simulink model "sm_forklift"  (R2026a)
settings: Solver=daessc  StopTime=stopTime
undefined symbols (not defined in the file): activeTestCmds, ForkliftParams, Ideal, X, Y, Z
libraries: sm_lib x153, nesl_utility x33, fl_lib x12, sm_forklift_lib x4, sdl_lib x3, Camera_Frame_Definitions x1, ee_lib x1, grid_element x1, simulink_extras x1, SignalEditorBlockLib x1
(part 1 of 7)
Description:
  | Copyright 2025-2026 The MathWorks, Inc.
settings Model: Creator=gabri  LastModifiedBy=smiller
settings DataIOCC: ExternalInput=[t,u]  SignalLoggingName=logsout_sm_forklift
settings SimscapeCC: SimscapeNominalValues="[{\"value\":\"1\",\"unit\":\"A\"},{\"value\":\"1\",\"unit\":\"bar\"},{\"value\":\"1\",\"unit\":\"cm^2\"},{\"value\":\"1\",\"unit\":\"cm^3/s\"},{\"value\":\"1\",\"unit\":\"kJ/kg\"},{\"value\":\"1\",\"unit\":\"kW\"},{\"value\":\"1\",\"unit\":\"l\"},{\"value\":\"1\",\"unit\":\"N\"},{\"value\":\"1\",\"unit\":\"N*m\"},{\"value\":\"1\",\"unit\":\"V\"}]"  SimscapeLogName=simlog_sm_forklift  SimscapeLogLimitData=off  SimscapeLogDataHistory=5000.0
settings DiagnosticsConfigSet: SimMechanicsConflictingReferenceFrames=none
settings ExplorerConfigSet: InternalSimMechanicsExplorerSettings="<ExplorerConfiguration><canonicalview>default</canonicalview><AnimationSetting><BasePlaybackSpeed>1.0</BasePlaybackSpeed><PlaybackSpeedFactor>2.0</PlaybackSpeedFactor></AnimationSetting><TilePanel><TileInfo><Tiles Columns=\"2\" Count=\"3\" Rows=\"2\"><Column Weight=\"0.5\"/><Column Weight=\"0.5\"/><Row Weight=\"0.4992\"/><Row Weight=\"0.5008\"/><Tile Height=\"2\" Width=\"1\" X=\"0\" Y=\"0\"/><Tile Height=\"1\" Width=\"1\" X=\"1\" Y=\"0\"/><Tile Height=\"1\" Width=\"1\" X=\"1\" Y=\"1\"/></Tiles></TileInfo><SceneInfo><SceneViewer><BGColor><R>1</R><G>1</G><B>1</B></BGColor><Camera><DoPerspective>on</DoPerspective><Position><X>4.09572120067952739</X><Y>-3.20098882363330972</Y><Z>2.29774941731300508</Z></Position><Center><X>3.34545211978248291</X><Y>-2.5757645895524397</Y><Z>2.08282858684770611</Z></Center><Up><X>-0.16510675539218278</X><Y>0.137588962826818928</Y><Z>0.976631474319820447</Z></Up><ViewLimDist>1</ViewLimDist><YLim>0.466307658154998583</YLim><XLim>0.48985854998100864</XLim></Camera></SceneViewer><SceneViewer><BGColor><R>1</R><G>1</G><B>1</B></BGColor><Camera><DoPerspective>on</DoPerspective><Position><X>0.255721200679526584</X><Y>-0.000988823633308211214</Y><Z>7.19774941731300544</Z></Position><Center><X>0.255721200679526584</X><Y>-0.000988823633308211214</Y><Z>6.19774941731300544</Z></Center><Up><X>0</X><Y>1</Y><Z>0</Z></Up><ViewLimDist>1</ViewLimDist><YLim>0.466307658154998583</YLim><XLim>0.996493077701092966</XLim></Camera></SceneViewer><SceneViewer><BGColor><R>1</R><G>1</G><B>1</B></BGColor><Camera><DoPerspective>on</DoPerspective><Position><X>0.255721200679527028</X><Y>-5.00098882363330866</Y><Z>1.8477494173130049</Z></Position><Center><X>0.255721200679526806</X><Y>-4.00933320629007106</Y><Z>1.71883418705838409</Z></Center><Up><X>-1.38777878078144568e-17</X><Y>0.128915230254620927</Y><Z>0.991655617343237816</Z></Up><ViewLimDist>1</ViewLimDist><YLim>0.466307658154998583</YLim><XLim>0.993092077435901444</XLim></Camera></SceneViewer></SceneInfo></TilePanel><MechEditorPanel><Cameras><Camera><Id>Camera1</Id><Value><Name>Track FixO FR</Name><NativeCamera><PositionTrackingFeature>Camera_Frames.Frame_FixO_FR.R</PositionTrackingFeature><CenterTrackingFeature>Camera_Frames.Frame_FixO_FR.R</CenterTrackingFeature><UpVectorTrackingFeature>Camera_Frames.Frame_FixO_FR.R</UpVectorTrackingFeature><CenterTrackingOrigin>off</CenterTrackingOrigin><CenterTrackingDirection>+X</CenterTrackingDirection><UpVectorTrackingDirection>+Z</UpVectorTrackingDirection></NativeCamera></Value></Camera><Camera><Id>Camera2</Id><Value><Name>Track FixO Right</Name><NativeCamera><PositionTrackingFeature>Camera_Frames.Frame_FixO_Right.R</PositionTrackingFeature><CenterTrackingFeature>Camera_Frames.Frame_FixO_Right.R</CenterTrackingFeature><UpVectorTrackingFeature>Camera_Frames.Frame_FixO_Right.R</UpVectorTrackingFeature><CenterTrackingOrigin>off</CenterTrackingOrigin><CenterTrackingDirection>+X</CenterTrackingDirection><UpVectorTrackingDirection>+Z</UpVectorTrackingDirection></NativeCamera></Value></Camera><Camera><Id>Camera3</Id><Value><Name>Track FixO RR</Name><NativeCamera><PositionTrackingFeature>Camera_Frames.Frame_FixO_RR.R</PositionTrackingFeature><CenterTrackingFeature>Camera_Frames.Frame_FixO_RR.R</CenterTrackingFeature><UpVectorTrackingFeature>Camera_Frames.Frame_FixO_RR.R</UpVectorTrackingFeature><CenterTrackingOrigin>off</CenterTrackingOrigin><CenterTrackingDirection>+X</CenterTrackingDirection><UpVectorTrackingDirection>+Z</UpVectorTrackingDirection></NativeCamera></Value></Camera><Camera><Id>Camera4</Id><Value><Name>Track FixO RL</Name><NativeCamera><PositionTrackingFeature>Camera_Frames.Frame_FixO_RL.R</PositionTrackingFeature><CenterTrackingFeature>Camera_Frames.Frame_FixO_RL.R</CenterTrackingFeature><UpVectorTrackingFeature>Camera_Frames.Frame_FixO_RL.R</UpVectorTrackingFeature><CenterTrackingOrigin>off</CenterTrackingOrigin><CenterTrackingDirection>+X</CenterTrackingDirection><UpVectorTrackingDirection>+Z</UpVectorTrackingDirection></NativeCamera></Value></Camera><Camera><Id>Camera5</Id><Value><Name>Track FixO Left</Name><NativeCamera><PositionTrackingFeature>Camera_Frames.Frame_FixO_Left.R</PositionTrackingFeature><CenterTrackingFeature>Camera_Frames.Frame_FixO_Left.R</CenterTrackingFeature><UpVectorTrackingFeature>Camera_Frames.Frame_FixO_Left.R</UpVectorTrackingFeature><CenterTrackingOrigin>off</CenterTrackingOrigin><CenterTrackingDirection>+X</CenterTrackingDirection><UpVectorTrackingDirection>+Z</UpVectorTrackingDirection></NativeCamera></Value></Camera><Camera><Id>Camera6</Id><Value><Name>Track FixO FL</Name><NativeCamera><PositionTrackingFeature>Camera_Frames.Frame_FixO_FL.R</PositionTrackingFeature><CenterTrackingFeature>Camera_Frames.Frame_FixO_FL.R</CenterTrackingFeature><UpVectorTrackingFeature>Camera_Frames.Frame_FixO_FL.R</UpVectorTrackingFeature><CenterTrackingOrigin>off</CenterTrackingOrigin><CenterTrackingDirection>+X</CenterTrackingDirection><UpVectorTrackingDirection>+Z</UpVectorTrackingDirection></NativeCamera></Value></Camera><Camera><Id>Camera7</Id><Value><Name>Track FixO Top</Name><NativeCamera><PositionTrackingFeature>Camera_Frames.Frame_FixO_Top.R</PositionTrackingFeature><CenterTrackingFeature>Camera_Frames.Frame_FixO_Top.R</CenterTrackingFeature><UpVectorTrackingFeature>Camera_Frames.Frame_FixO_Top.R</UpVectorTrackingFeature><CenterTrackingOrigin>off</CenterTrackingOrigin><CenterTrackingDirection>+X</CenterTrackingDirection><UpVectorTrackingDirection>+Z</UpVectorTrackingDirection></NativeCamera></Value></Camera><Camera><Id>Camera8</Id><Value><Name>Track FixO Front</Name><NativeCamera><PositionTrackingFeature>Camera_Frames.Frame_FixO_Front.R</PositionTrackingFeature><CenterTrackingFeature>Camera_Frames.Frame_FixO_Front.R</CenterTrackingFeature><UpVectorTrackingFeature>Camera_Frames.Frame_FixO_Front.R</UpVectorTrackingFeature><CenterTrackingOrigin>off</CenterTrackingOrigin><CenterTrackingDirection>+X</CenterTrackingDirection><UpVectorTrackingDirection>+Z</UpVectorTrackingDirection></NativeCamera></Value></Camera><Camera><Id>Camera9</Id><Value><Name>Track FixO Rear</Name><NativeCamera><PositionTrackingFeature>Camera_Frames.Frame_FixO_Rear.R</PositionTrackingFeature><CenterTrackingFeature>Camera_Frames.Frame_FixO_Rear.R</CenterTrackingFeature><UpVectorTrackingFeature>Camera_Frames.Frame_FixO_Rear.R</UpVectorTrackingFeature><CenterTrackingOrigin>off</CenterTrackingOrigin><CenterTrackingDirection>+X</CenterTrackingDirection><UpVectorTrackingDirection>+Z</UpVectorTrackingDirection></NativeCamera></Value></Camera><Camera><Id>Camera10</Id><Value><Name>Track FR</Name><NativeCamera><PositionTrackingFeature>Camera_Frames.Frame_FR.R</PositionTrackingFeature><CenterTrackingFeature>Camera_Frames.Frame_FR.R</CenterTrackingFeature><UpVectorTrackingFeature>Camera_Frames.Frame_FR.R</UpVectorTrackingFeature><CenterTrackingOrigin>off</CenterTrackingOrigin><CenterTrackingDirection>+X</CenterTrackingDirection><UpVectorTrackingDirection>+Z</UpVectorTrackingDirection></NativeCamera></Value></Camera><Camera><Id>Camera11</Id><Value><Name>Track Right</Name><NativeCamera><PositionTrackingFeature>Camera_Frames.Frame_Right.R</PositionTrackingFeature><CenterTrackingFeature>Camera_Frames.Frame_Right.R</CenterTrackingFeature><UpVectorTrackingFeature>Camera_Frames.Frame_Right.R</UpVectorTrackingFeature><CenterTrackingOrigin>off</CenterTrackingOrigin><CenterTrackingDirection>+X</CenterTrackingDirection><UpVectorTrackingDirection>+Z</UpVectorTrackingDirection></NativeCamera></Value></Camera><Camera><Id>Camera12</Id><Value><Name>Track RR</Name><NativeCamera><PositionTrackingFeature>Camera_Frames.Frame_RR.R</PositionTrackingFeature><CenterTrackingFeature>Camera_Frames.Frame_RR.R</CenterTrackingFeature><UpVectorTrackingFeature>Camera_Frames.Frame_RR.R</UpVectorTrackingFeature><CenterTrackingOrigin>off</CenterTrackingOrigin><CenterTrackingDirection>+X</CenterTrackingDirection><UpVectorTrackingDirection>+Z</UpVectorTrackingDirection></NativeCamera></Value></Camera><Camera><Id>Camera13</Id><Value><Name>Track RL</Name><NativeCamera><PositionTrackingFeature>Camera_Frames.Frame_RL.R</PositionTrackingFeature><CenterTrackingFeature>Camera_Frames.Frame_RL.R</CenterTrackingFeature><UpVectorTrackingFeature>Camera_Frames.Frame_RL.R</UpVectorTrackingFeature><CenterTrackingOrigin>off</CenterTrackingOrigin><CenterTrackingDirection>+X</CenterTrackingDirection><UpVectorTrackingDirection>+Z</UpVectorTrackingDirection></NativeCamera></Value></Camera><Camera><Id>Camera14</Id><Value><Name>Track Left</Name><NativeCamera><PositionTrackingFeature>Camera_Frames.Frame_Left.R</PositionTrackingFeature><CenterTrackingFeature>Camera_Frames.Frame_Left.R</CenterTrackingFeature><UpVectorTrackingFeature>Camera_Frames.Frame_Left.R</UpVectorTrackingFeature><CenterTrackingOrigin>off</CenterTrackingOrigin><CenterTrackingDirection>+X</CenterTrackingDirection><UpVectorTrackingDirection>+Z</UpVectorTrackingDirection></NativeCamera></Value></Camera><Camera><Id>Camera15</Id><Value><Name>Track FL</Name><NativeCamera><PositionTrackingFeature>Camera_Frames.Frame_FL.R</PositionTrackingFeature><CenterTrackingFeature>Camera_Frames.Frame_FL.R</CenterTrackingFeature><UpVectorTrackingFeature>Camera_Frames.Frame_FL.R</UpVectorTrackingFeature><CenterTrackingOrigin>off</CenterTrackingOrigin><CenterTrackingDirection>+X</CenterTrackingDirection><UpVectorTrackingDirection>+Z</UpVectorTrackingDirection></NativeCamera></Value></Camera><Camera><Id>Camera16</Id><Value><Name>Track Top</Name><NativeCamera><PositionTrackingFeature>Camera_Frames.Frame_Top.R</PositionTrackingFeature><CenterTrackingFeature>Camera_Frames.Frame_Top.R</CenterTrackingFeature><UpVectorTrackingFeature>Camera_Frames.Frame_Top.R</UpVectorTrackingFeature><CenterTrackingOrigin>off</CenterTrackingOrigin><CenterTrackingDirection>+X</CenterTrackingDirection><UpVectorTrackingDirection>+Z</UpVectorTrackingDirection></NativeCamera></Value></Camera><Camera><Id>Camera17</Id><Value><Name>Track Front</Name><NativeCamera><PositionTrackingFeature>Camera_Frames.Frame_Front.R</PositionTrackingFeature><CenterTrackingFeature>Camera_Frames.Frame_Front.R</CenterTrackingFeature><UpVectorTrackingFeature>Camera_Frames.Frame_Front.R</UpVectorTrackingFeature><CenterTrackingOrigin>off</CenterTrackingOrigin><CenterTrackingDirection>+X</CenterTrackingDirection><UpVectorTrackingDirection>+Z</UpVectorTrackingDirection></NativeCamera></Value></Camera><Camera><Id>Camera18</Id><Value><Name>Track Rear</Name><NativeCamera><PositionTrackingFeature>Camera_Frames.Frame_Rear.R</PositionTrackingFeature><CenterTrackingFeature>Camera_Frames.Frame_Rear.R</CenterTrackingFeature><UpVectorTrackingFeature>Camera_Frames.Frame_Rear.R</UpVectorTrackingFeature><CenterTrackingOrigin>off</CenterTrackingOrigin><CenterTrackingDirection>+X</CenterTrackingDirection><UpVectorTrackingDirection>+Z</UpVectorTrackingDirection></NativeCamera></Value></Camera><Camera><Id>Camera19</Id><Value><Name>Track SuspF</Name><NativeCamera><PositionTrackingFeature>Camera_Frames.Frame_SuspF.R</PositionTrackingFeature><CenterTrackingFeature>Camera_Frames.Frame_SuspF.R</CenterTrackingFeature><UpVectorTrackingFeature>Camera_Frames.Frame_SuspF.R</UpVectorTrackingFeature><CenterTrackingOrigin>off</CenterTrackingOrigin><CenterTrackingDirection>+X</CenterTrackingDirection><UpVectorTrackingDirection>+Z</UpVectorTrackingDirection></NativeCamera></Value></Camera><Camera><Id>Camera20</Id><Value><Name>Track SuspR</Name><NativeCamera><PositionTrackingFeature>Camera_Frames.Frame_SuspR.R</PositionTrackingFeature><CenterTrackingFeature>Camera_Frames.Frame_SuspR.R</CenterTrackingFeature><UpVectorTrackingFeature>Camera_Frames.Frame_SuspR.R</UpVectorTrackingFeature><CenterTrackingOrigin>off</CenterTrackingOrigin><CenterTrackingDirection>+X</CenterTrackingDirection><UpVectorTrackingDirection>+Z</UpVectorTrackingDirection></NativeCamera></Value></Camera><Camera><Id>Camera21</Id><Value><Name>Track WheelFR</Name><NativeCamera><PositionTrackingFeature>Camera_Frames.Frame_Wheel_FR.R</PositionTrackingFeature><CenterTrackingFeature>Camera_Frames.Frame_Wheel_FR.R</CenterTrackingFeature><UpVectorTrackingFeature>Camera_Frames.Frame_Wheel_FR.R</UpVectorTrackingFeature><CenterTrackingOrigin>off</CenterTrackingOrigin><CenterTrackingDirection>+X</CenterTrackingDirection><UpVectorTrackingDirection>+Z</UpVectorTrackingDirection></NativeCamera></Value></Camera><Camera><Id>Camera22</Id><Value><Name>Track WheelRR</Name><NativeCamera><PositionTrackingFeature>Camera_Frames.Frame_Wheel_RR.R</PositionTrackingFeature><CenterTrackingFeature>Camera_Frames.Frame_Wheel_RR.R</CenterTrackingFeature><UpVectorTrackingFeature>Camera_Frames.Frame_Wheel_RR.R</UpVectorTrackingFeature><CenterTrackingOrigin>off</CenterTrackingOrigin><CenterTrackingDirection>+X</CenterTrackingDirection><UpVectorTrackingDirection>+Z</UpVectorTrackingDirection></NativeCamera></Value></Camera><Camera><Id>Camera23</Id><Value><Name>Track WheelRL</Name><NativeCamera><PositionTrackingFeature>Camera_Frames.Frame_Wheel_RL.R</PositionTrackingFeature><CenterTrackingFeature>Camera_Frames.Frame_Wheel_RL.R</CenterTrackingFeature><UpVectorTrackingFeature>Camera_Frames.Frame_Wheel_RL.R</UpVectorTrackingFeature><CenterTrackingOrigin>off</CenterTrackingOrigin><CenterTrackingDirection>+X</CenterTrackingDirection><UpVectorTrackingDirection>+Z</UpVectorTrackingDirection></NativeCamera></Value></Camera><Camera><Id>Camera24</Id><Value><Name>Track WheelFL</Name><NativeCamera><PositionTrackingFeature>Camera_Frames.Frame_Wheel_FL.R</PositionTrackingFeature><CenterTrackingFeature>Camera_Frames.Frame_Wheel_FL.R</CenterTrackingFeature><UpVectorTrackingFeature>Camera_Frames.Frame_Wheel_FL.R</UpVectorTrackingFeature><CenterTrackingOrigin>off</CenterTrackingOrigin><CenterTrackingDirection>+X</CenterTrackingDirection><UpVectorTrackingDirection>+Z</UpVectorTrackingDirection></NativeCamera></Value></Camera><Camera><Id>Camera25</Id><Value><Name>View Seat FL</Name><NativeCamera><PositionTrackingFeature>Camera_Frames.Frame_View_Seat_FL.R</PositionTrackingFeature><CenterTrackingFeature>Camera_Frames.Frame_View_Seat_FL.R</CenterTrackingFeature><UpVectorTrackingFeature>Camera_Frames.Frame_View_Seat_FL.R</UpVectorTrackingFeature><CenterTrackingOrigin>off</CenterTrackingOrigin><CenterTrackingDirection>+X</CenterTrackingDirection><UpVectorTrackingDirection>+Z</UpVectorTrackingDirection></NativeCamera></Value></Camera><Camera><Id>Camera26</Id><Value><Name>View Seat FR</Name><NativeCamera><PositionTrackingFeature>Camera_Frames.Frame_View_Seat_FR.R</PositionTrackingFeature><CenterTrackingFeature>Camera_Frames.Frame_View_Seat_FR.R</CenterTrackingFeature><UpVectorTrackingFeature>Camera_Frames.Frame_View_Seat_FR.R</UpVectorTrackingFeature><CenterTrackingOrigin>off</CenterTrackingOrigin><CenterTrackingDirection>+X</CenterTrackingDirection><UpVectorTrackingDirection>+Z</UpVectorTrackingDirection></NativeCamera></Value></Camera><Camera><Id>Camera27</Id><Value><Name>View Susp FR</Name><NativeCamera><PositionTrackingFeature>Camera_Frames.Frame_View_Susp_FR.R</PositionTrackingFeature><CenterTrackingFeature>Camera_Frames.Frame_View_Susp_FR.R</CenterTrackingFeature><UpVectorTrackingFeature>Camera_Frames.Frame_View_Susp_FR.R</UpVectorTrackingFeature><CenterTrackingOrigin>off</CenterTrackingOrigin><CenterTrackingDirection>+X</CenterTrackingDirection><UpVectorTrackingDirection>+Z</UpVectorTrackingDirection></NativeCamera></Value></Camera><Camera><Id>Camera28</Id><Value><Name>View Susp RR</Name><NativeCamera><PositionTrackingFeature>Camera_Frames.Frame_View_Susp_RR.R</PositionTrackingFeature><CenterTrackingFeature>Camera_Frames.Frame_View_Susp_RR.R</CenterTrackingFeature><UpVectorTrackingFeature>Camera_Frames.Frame_View_Susp_RR.R</UpVectorTrackingFeature><CenterTrackingOrigin>off</CenterTrackingOrigin><CenterTrackingDirection>+X</CenterTrackingDirection><UpVectorTrackingDirection>+Z</UpVectorTrackingDirection></NativeCamera></Value></Camera><Camera><Id>Camera29</Id><Value><Name>View Susp RL</Name><NativeCamera><PositionTrackingFeature>Camera_Frames.Frame_View_Susp_RL.R</PositionTrackingFeature><CenterTrackingFeature>Camera_Frames.Frame_View_Susp_RL.R</CenterTrackingFeature><UpVectorTrackingFeature>Camera_Frames.Frame_View_Susp_RL.R</UpVectorTrackingFeature><CenterTrackingOrigin>off</CenterTrackingOrigin><CenterTrackingDirection>+X</CenterTrackingDirection><UpVectorTrackingDirection>+Z</UpVectorTrackingDirection></NativeCamera></Value></Camera><Camera><Id>Camera30</Id><Value><Name>View Susp FL</Name><NativeCamera><PositionTrackingFeature>Camera_Frames.Frame_View_Susp_FL.R</PositionTrackingFeature><CenterTrackingFeature>Camera_Frames.Frame_View_Susp_FL.R</CenterTrackingFeature><UpVectorTrackingFeature>Camera_Frames.Frame_View_Susp_FL.R</UpVectorTrackingFeature><CenterTrackingOrigin>off</CenterTrackingOrigin><CenterTrackingDirection>+X</CenterTrackingDirection><UpVectorTrackingDirection>+Z</UpVectorTrackingDirection></NativeCamera></Value></Camera><Camera><Id>Camera31</Id><Value><Name>Dolly Camera</Name><NativeCamera><PositionTrackingFeature>Camera_Frames.Frame_Dolly.R</PositionTrackingFeature><CenterTrackingFeature>Camera_Frames.Frame_Dolly.R</CenterTrackingFeature><UpVectorTrackingFeature>Camera_Frames.Frame_Dolly.R</UpVectorTrackingFeature><CenterTrackingOrigin>off</CenterTrackingOrigin><CenterTrackingDirection>+X</CenterTrackingDirection><UpVectorTrackingDirection>+Z</UpVectorTrackingDirection></NativeCamera></Value></Camera><Camera><Id>Camera32</Id><Value><Name>Track Dolly Camera</Name><NativeCamera><PositionTrackingFeature>Camera_Frames.Frame_Dolly.R</PositionTrackingFeature><CenterTrackingFeature>Camera_Frames.Transform_Camera_Ref.F</CenterTrackingFeature><UpVectorTrackingFeature>Camera_Frames.World_Frame.W</UpVectorTrackingFeature><CenterTrackingOrigin>on</CenterTrackingOrigin><UpVectorTrackingDirection>+Z</UpVectorTrackingDirection></NativeCamera></Value></Camera></Cameras><GfxPanelCameraMap><MapElement CameraMLId=\"Camera1\" GfxPanelIndex=\"0\"/><MapElement CameraMLId=\"Camera7\" GfxPanelIndex=\"1\"/><MapElement CameraMLId=\"Camera2\" GfxPanelIndex=\"2\"/></GfxPanelCameraMap><VideoCreator><PlaybackSpeedRatio>1.0</PlaybackSpeedRatio><FrameRate>30</FrameRate><VideoFormat>MPEG-4</VideoFormat><FrameSize>[800 450]</FrameSize></VideoCreator></MechEditorPanel></ExplorerConfiguration>"

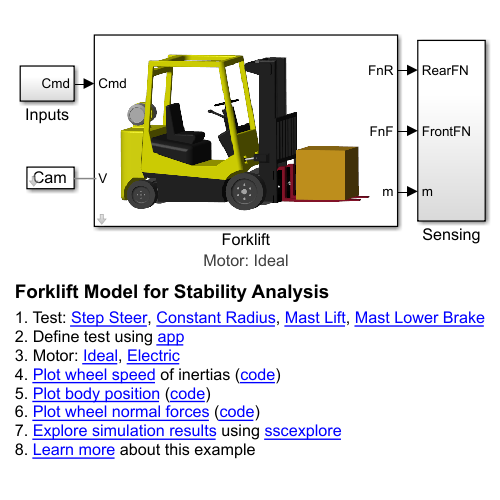
[thumbnail: Simulink's stored preview of the top-level diagram]
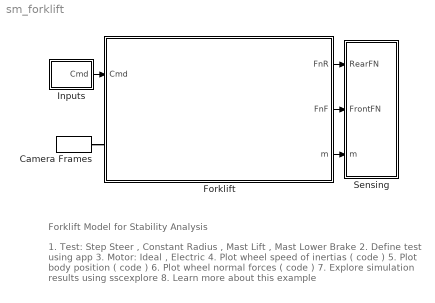
== system sm_forklift ==
  note: 1. Test: Step Steer , Constant Radius , Mast Lift , Mast Lower Brake
      | 2. Define test using app
      | 3. Motor: Ideal , Electric
      | 4. Plot wheel speed of inertias ( code )
      | 5. Plot body position ( code )
      | 6. Plot wheel normal forces ( code )
      | 7. Explore simulation results using sscexplore
      | 8. Learn more about this example
  note: Forklift Model for Stability Analysis
  Camera Frames : Camera_Frame_Definitions/Camera Frames  Camera=Camera  popup_dolly_camera=XYZ
  Forklift : Subsystem  mask{popup_motor_type=Ideal, popup_fnVis_onOff=On}
      mask prompts: popup_motor_type "Motor Type"; popup_fnVis_onOff "Normal Force Visualization"
      settings: AttributesFormatString=Motor: %<popup_motor_type>
      mask TypeOptions popup_motor_type: AxleF/popup_motor_type
      mask TypeOptions popup_fnVis_onOff: AxleR/popup_fnVis_onOff | AxleF/popup_fnVis_onOff
      mask Display: image('sm_forklift_full_image.png');
  Inputs : Subsystem
  Sensing : Subsystem
  wires:
  Forklift/1(FnR) -> Sensing/1(RearFN)
  Forklift/2(FnF) -> Sensing/2(FrontFN)
  Forklift/3(m) -> Sensing/3(m)
  Inputs/1(Cmd) -> Forklift/1(Cmd)
  connections:
  Camera Frames/RConn1 -- Forklift/LConn1

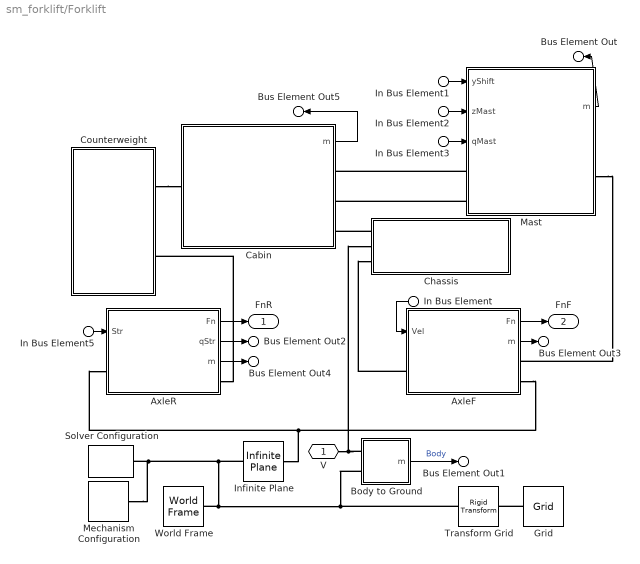
== system sm_forklift/Forklift ==
  In Bus Element : Inport  PortName=Cmd  Element=vVeh
  In Bus Element1 : Inport  PortName=Cmd  Element=yShift
  In Bus Element2 : Inport  PortName=Cmd  Element=zMast
  In Bus Element3 : Inport  PortName=Cmd  Element=qTilt
  In Bus Element5 : Inport  PortName=Cmd  Element=qStr
  AxleF : Subsystem  mask{popup_motor_type=Ideal, popup_fnVis_onOff=On}
      mask prompts: popup_motor_type "Motor Type"; popup_fnVis_onOff "Normal Force Visualization"
      settings: AttributesFormatString=%<popup_motor_type>
      mask TypeOptions popup_motor_type: Motor/popup_motor_type
      mask TypeOptions popup_fnVis_onOff: Vis Fn L/popup_fnVis_onOff | Vis Fn R/popup_fnVis_onOff
      mask Display: image('sm_forklift_axlef_image.png')
  AxleR : Subsystem  mask{popup_fnVis_onOff=On}
      mask prompts: popup_fnVis_onOff "Normal Force Visualization"
      mask TypeOptions popup_fnVis_onOff: Vis Fn L/popup_fnVis_onOff | Vis Fn R/popup_fnVis_onOff
      mask Display: image('sm_forklift_axler_image.png');
  Body to Ground : Subsystem
  Cabin : Subsystem
      mask Display: image('sm_forklift_cabin_image.png');
  Chassis : Subsystem
      mask Display: image('sm_forklift_chassis_image.png');
  Counterweight : Subsystem
      mask Display: image('sm_forklift_counterweight_image.png')
  Grid : grid_element/Grid  VariantControl=Grid  grid_x=3*6*4  grid_y=4*4  grid_z=0.02  grid_line_width=0.02  grid_num_sq_x=3*6*2  grid_num_sq_y=4*2  grid_offset=[25 0 0]  grid_clr=[1 1 1]  plane_clr=[1 1 1]  grid_opc=1  plane_opc=1
  Infinite Plane : sm_lib/Curves and Surfaces/Infinite Plane  GraphicType=None  GraphicPlaneWidth=1  GraphicPlaneWidthUnits=m  GraphicPlaneHeight=1  GraphicPlaneHeightUnits=m  GraphicVisPropType=SimpleVisualProperties  GraphicDiffuseColor=[0.5 0.5 0.5]  GraphicOpacity=1  GraphicSpecularColor=[0.5 0.5 0.5 1.0]  GraphicAmbientColor=[0.15 0.15 0.15 1.0]  GraphicEmissiveColor=[0.0 0.0 0.0 1.0]  GraphicShininess=75
  Mast : Subsystem
      mask Display: image('sm_forklift_mast_image.png');
  Mechanism Configuration : sm_lib/Utilities/Mechanism Configuration  UniformGravity=Constant  GravityVector=[0 0 -9.80665]  GravityVectorUnits=m/s^2  LinearizationDelta=0.001  JointModeTransitionNonlinearIterations=2
  Solver Configuration : nesl_utility/Solver Configuration  PhysicalDomain=network_engine_domain  SubClassName=solver  LeftPortType=input  RightPortType=generic  Tones=[]  Harmonics=[]  SimulateNoise=off  Profile=off  UseLocalSampling=off  EnableSwitchedLinearOptims=on  FrequencyDomain=off  UseCCode=off  RelTol=0.001  AbsTol=0.001  MinStep=1e-09  ToWorkspace=off  RevertToSquareIcSolve=off  NumHomotopyIterations=100  PhasorMode=off  PhasorModeNumHarmonics=1  ConsistencySolver=NEWTON_XTOL_AFTER_FTOL  CanonicalOrdering=UNORDERED  OptimizeIntermediates=UNOPTIMIZED  IndexReductionMethod=DerivativeReplacement  DoDC=off  ResidualTolerance=1e-09  ConsistencyTolSource=GLOBAL  ConsistencyAbsTol=0.001  ConsistencyRelTol=0.001  ConsistencyTolFactor=0.001  UseLocalSolver=off  LocalSolverChoice=NE_BACKWARD_EULER_ADVANCER  ResolveIndetEquations=on  FunctionEvalNumThread=1  LocalSolverSampleTime=0.001  DoFixedCost=off  MaxNonlinIter=3  MaxModeIter=2  ComputeImpulses=off  ImpulseIterations=2  LinearAlgebra=auto  LinearAlgebraNumThread=0  EquationFormulation=NE_TIME_EF  DelaysMemoryBudget=1024  AutomaticFiltering=on  FilteringTimeConstant=0.001  PartitionStorageMethod=AS_NEEDED  PartitionMemoryBudget=1024  PartitionMethod=ROBUST  MultibodyUseLocalSolver=off  MultibodyLocalSolverChoice=ODE1  MultibodyLocalSolverSampleTime=0.001
  Transform Grid : sm_lib/Frames and Transforms/Rigid Transform  RotationMethod=None  FollAlignAxisA=+X  BaseAlignAxisA=+Y  FollAlignAxisB=+Y  BaseAlignAxisB=+Z  RotationStandardAxis=+Z  RotationAngle=0  RotationAngleUnits=deg  RotationArbitraryAxis=[0 0 1]  RotationSequenceAxes=FollowerAxes  RotationSequence=XYX  RotationSequenceAngles=[0 0 0]  RotationSequenceAnglesUnits=deg  RotationMatrix=[1 0 0;0 1 0;0 0 1]  Quaternion=[1 0 0 0]  TranslationMethod=None  TranslationCartesianOffset=[0 0 0]  TranslationCartesianOffsetUnits=m  TranslationStandardAxis=+Z  TranslationStandardOffset=0  TranslationStandardOffsetUnits=m  TranslationROffset=0  TranslationROffsetUnits=m  TranslationThetaOffset=0  TranslationThetaOffsetUnits=deg  TranslationZOffset=0  TranslationZOffsetUnits=m
  World Frame : sm_lib/Frames and Transforms/World Frame
  V : PMIOPort  Side=Left
  FnR : Outport
  FnF : Outport  Port=2
  Bus Element Out : Outport  Port=3  PortName=m  Element=Mast
  Bus Element Out1 : Outport  Port=3  PortName=m  Element=Body
  Bus Element Out2 : Outport  Port=3  PortName=m  Element=SteerAngle
  Bus Element Out3 : Outport  Port=3  PortName=m  Element=AxleF
  Bus Element Out4 : Outport  Port=3  PortName=m  Element=AxleR
  Bus Element Out5 : Outport  Port=3  PortName=m  Element=Cabin
  wires:
  In Bus Element/1 -> AxleF/1(Vel)
  AxleF/1(Fn) -> FnF/1
  AxleR/1(Fn) -> FnR/1
  In Bus Element5/1 -> AxleR/1(Str)
  In Bus Element3/1 -> Mast/3(qMast)
  In Bus Element1/1 -> Mast/1(yShift)
  In Bus Element2/1 -> Mast/2(zMast)
  AxleR/2(qStr) -> Bus Element Out2/1
  Mast/1(m) -> Bus Element Out/1
  Body to Ground/1(m) -> Bus Element Out1/1  "Body"
  AxleF/2(m) -> Bus Element Out3/1
  AxleR/3(m) -> Bus Element Out4/1
  Cabin/1(m) -> Bus Element Out5/1
  connections:
  Infinite Plane/RConn1 -- AxleF/RConn2 -- AxleR/LConn1
  AxleR/RConn1 -- Counterweight/RConn2
  Infinite Plane/LConn1 -- Mechanism Configuration/RConn1 -- Solver Configuration/RConn1 -- Body to Ground/LConn2 -- Transform Grid/LConn1 -- World Frame/RConn1
  Mast/LConn1 -- Cabin/RConn1
  Counterweight/RConn1 -- Cabin/LConn1
  Mast/RConn1 -- AxleF/RConn1
  Mast/LConn2 -- Cabin/RConn2
  Chassis/LConn1 -- Cabin/RConn3
  AxleF/LConn1 -- Chassis/LConn3
  Body to Ground/LConn1 -- V/RConn1 -- Chassis/LConn2
  Grid/RConn1 -- Transform Grid/RConn1

== system sm_forklift/Inputs ==
  Bus Creator1 : BusCreator  Inputs=5
  Clock : Clock
  Command Lift : Lookup_n-D  NumberOfTableDimensions=1  BreakpointsForDimension1=activeTestCmds.get('MastLiftPos').Time  Table=activeTestCmds.get('MastLiftPos').Data  InternalRulePriority=Speed  RndMeth=Simplest
  Command Shift : Lookup_n-D  NumberOfTableDimensions=1  BreakpointsForDimension1=activeTestCmds.get('SideShiftPos').Time  Table=activeTestCmds.get('SideShiftPos').Data  InternalRulePriority=Speed  RndMeth=Simplest
  Command Steer : Lookup_n-D  NumberOfTableDimensions=1  BreakpointsForDimension1=activeTestCmds.get('SteerAngle').Time  Table=activeTestCmds.get('SteerAngle').Data  InternalRulePriority=Speed  RndMeth=Simplest
  Command Tilt : Lookup_n-D  NumberOfTableDimensions=1  BreakpointsForDimension1=activeTestCmds.get('MastTiltAngle').Time  Table=activeTestCmds.get('MastTiltAngle').Data  InternalRulePriority=Speed  RndMeth=Simplest
  Command Vel : Lookup_n-D  NumberOfTableDimensions=1  BreakpointsForDimension1=activeTestCmds.get('Velocity').Time  Table=activeTestCmds.get('Velocity').Data  InternalRulePriority=Speed  RndMeth=Simplest
  Signal Editor : SignalEditorBlockLib/Signal Editor  Commented=on  FileName=ForkliftTestCommands.mat  ActiveScenario=TestCmds  ActiveSignal=Velocity  IsBus=off  OutputBusObjectStr=Bus: BusObject  SampleTime=0  Interpolate=off  ZeroCross=off  OutputAfterFinalValue=Setting to zero  Unit=inherit  PreserveSignalName=on  ApplySigPropsToAllScenarios=on  ApplySigPropsToAllSignals=off  SignalPropertySource=Dialog parameters
  Cmd : Outport
  wires:
  Command Lift/1 -> Bus Creator1/2  "zMast"
  Command Tilt/1 -> Bus Creator1/3  "qTilt"
  Command Steer/1 -> Bus Creator1/4  "qStr"
  Bus Creator1/1 -> Cmd/1
  Clock/1 -> Command Lift/1, Command Shift/1, Command Steer/1, Command Tilt/1, Command Vel/1
  Command Shift/1 -> Bus Creator1/5  "yShift"
  Command Vel/1 -> Bus Creator1/1  "vVeh"

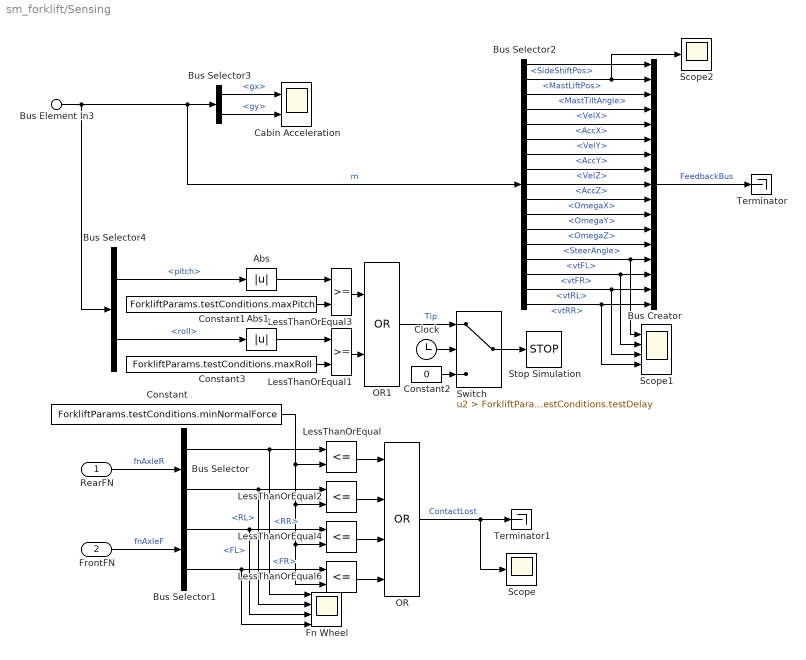
== system sm_forklift/Sensing ==
  RearFN : Inport
  FrontFN : Inport  Port=2
  Bus Element In3 : Inport  Port=3  PortName=m
  Abs : Abs  ZeroCross=off  SaturateOnIntegerOverflow=off
  Abs1 : Abs  ZeroCross=off  SaturateOnIntegerOverflow=off
  Bus Creator : BusCreator  Inputs=17
  Bus Selector : BusSelector  OutputSignals=RR,RL
  Bus Selector1 : BusSelector  OutputSignals=FL,FR
  Bus Selector2 : BusSelector  OutputSignals=Mast.SideShiftPos,Mast.MastLiftPos,Mast.MastTiltAngle,Body.VelX,Body.AccX,Body.VelY,Body.AccY,Body.VelZ,Body.AccZ,Body.OmegaX,Body.OmegaY,Body.OmegaZ,SteerAngle,AxleF.vtFL,AxleF.vtFR,AxleR.vtRL,AxleR.vtRR
  Bus Selector3 : BusSelector  OutputSignals=Cabin.gx,Cabin.gy
  Bus Selector4 : BusSelector  OutputSignals=Body.pitch,Body.roll
  Cabin Acceleration : Scope  NumInputPorts=2
      settings: ActiveDisplayYMinimum=-1.35728  ActiveDisplayYMaximum=6.28668  DataLoggingVariableName=ScopeData2
  Clock : Clock
  Constant : Constant  Value=ForkliftParams.testConditions.minNormalForce
  Constant1 : Constant  Value=ForkliftParams.testConditions.maxPitch
  Constant2 : Constant  Value=0
  Constant3 : Constant  Value=ForkliftParams.testConditions.maxRoll
  Fn Wheel : Scope  NumInputPorts=4
      settings: ActiveDisplayYMinimum=-5612.2162  ActiveDisplayYMaximum=50509.9458
  LessThanOrEqual{,2,4,6} (4 alike) : RelationalOperator  Operator=<=  OutDataTypeStr=boolean  RndMeth=Simplest  InputSameDT=off
  LessThanOrEqual1 : RelationalOperator  OutDataTypeStr=boolean  RndMeth=Simplest  InputSameDT=off
  LessThanOrEqual3 : RelationalOperator  OutDataTypeStr=boolean  RndMeth=Simplest  InputSameDT=off
  OR : Logic  Operator=OR  Inputs=4  IconShape=distinctive  AllPortsSameDT=off  OutDataTypeStr=boolean
  OR1 : Logic  Operator=OR  IconShape=distinctive  AllPortsSameDT=off  OutDataTypeStr=boolean
  Scope : Scope
      settings: ActiveDisplayYMinimum=-0.125  ActiveDisplayYMaximum=1.125  DataLoggingVariableName=ScopeData2
  Scope1 : Scope  NumInputPorts=4
      settings: ActiveDisplayYMinimum=-0.06302  ActiveDisplayYMaximum=0.56714
  Scope2 : Scope
      settings: ActiveDisplayYMinimum=4742.86133  ActiveDisplayYMaximum=4823.87254
  Stop Simulation : Stop
  Switch : Switch  Criteria=u2 > Threshold  Threshold=ForkliftParams.testConditions.testDelay  SaturateOnIntegerOverflow=off  InputSameDT=off
  Terminator : Terminator
  Terminator1 : Terminator
  wires:
  RearFN/1 -> Bus Selector/1  "fnAxleR"
  FrontFN/1 -> Bus Selector1/1  "fnAxleF"
  Constant/1 -> LessThanOrEqual6/2, LessThanOrEqual4/2, LessThanOrEqual2/2, LessThanOrEqual/2
  Bus Selector/1 -> LessThanOrEqual/1, Fn Wheel/1  "<RR>"
  Bus Selector/2 -> Fn Wheel/2, LessThanOrEqual2/1  "<RL>"
  LessThanOrEqual/1 -> OR/1
  LessThanOrEqual2/1 -> OR/2
  LessThanOrEqual6/1 -> OR/4
  LessThanOrEqual4/1 -> OR/3
  Bus Selector1/2 -> LessThanOrEqual6/1, Fn Wheel/4  "<FR>"
  Bus Selector1/1 -> LessThanOrEqual4/1, Fn Wheel/3  "<FL>"
  OR/1 -> Terminator1/1, Scope/1  "ContactLost"
  Bus Creator/1 -> Terminator/1  "FeedbackBus"
  Clock/1 -> Switch/2
  Constant2/1 -> Switch/3
  Bus Selector2/1 -> Bus Creator/1  "<SideShiftPos>"
  Bus Selector2/2 -> Scope2/1, Bus Creator/2  "<MastLiftPos>"
  Bus Selector2/3 -> Bus Creator/3  "<MastTiltAngle>"
  Bus Selector2/4 -> Bus Creator/4  "<VelX>"
  Bus Selector2/5 -> Bus Creator/5  "<AccX>"
  Bus Selector2/6 -> Bus Creator/6  "<VelY>"
  Bus Selector2/7 -> Bus Creator/7  "<AccY>"
  Bus Selector2/8 -> Bus Creator/8  "<VelZ>"
  Bus Selector2/9 -> Bus Creator/9  "<AccZ>"
  Bus Selector2/10 -> Bus Creator/10  "<OmegaX>"
  Bus Selector2/11 -> Bus Creator/11  "<OmegaY>"
  Bus Selector2/12 -> Bus Creator/12  "<OmegaZ>"
  Bus Selector2/13 -> Bus Creator/13  "<SteerAngle>"
  Bus Element In3/1 -> Bus Selector2/1, Bus Selector3/1, Bus Selector4/1  "m"
  Bus Selector2/14 -> Scope1/1, Bus Creator/14  "<vtFL>"
  Bus Selector2/15 -> Scope1/2, Bus Creator/15  "<vtFR>"
  Bus Selector2/16 -> Scope1/3, Bus Creator/16  "<vtRL>"
  Bus Selector2/17 -> Scope1/4, Bus Creator/17  "<vtRR>"
  Bus Selector3/1 -> Cabin Acceleration/1  "<gx>"
  Bus Selector3/2 -> Cabin Acceleration/2  "<gy>"
  Switch/1 -> Stop Simulation/1
  Bus Selector4/1 -> Abs/1  "<pitch>"
  Abs/1 -> LessThanOrEqual3/1
  Constant1/1 -> LessThanOrEqual3/2
  Bus Selector4/2 -> Abs1/1  "<roll>"
  Abs1/1 -> LessThanOrEqual1/1
  Constant3/1 -> LessThanOrEqual1/2
  LessThanOrEqual3/1 -> OR1/1
  LessThanOrEqual1/1 -> OR1/2
  OR1/1 -> Switch/1  "Tip"

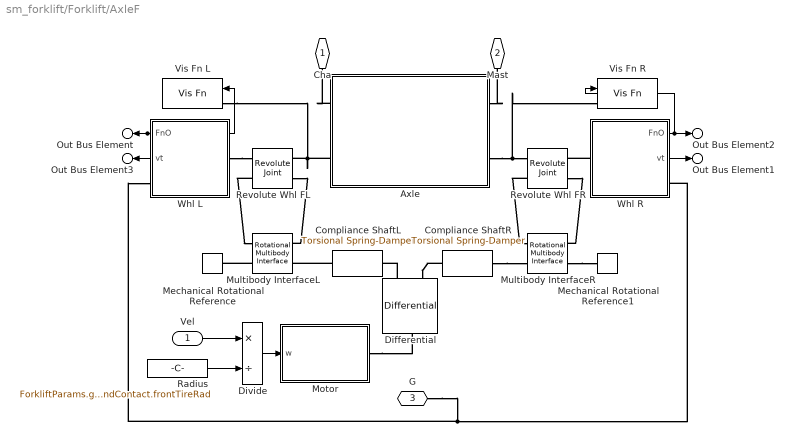
== system sm_forklift/Forklift/AxleF ==
  Vel : Inport
  Axle : Subsystem
      mask Display: image('sm_forklift_axleHousingF_image.png')
  Compliance ShaftL : sdl_lib/Couplings & Drives/Torsional Spring-Damper  k=1000*100 N*m/rad  mu_visc=1e3*10 N*m*s/rad  trq_coulomb=0 N*m  static_kinetic_ratio=1.1  w_tol=0.001 rad/s  model_hardstop=sdl.enum.hardStopOffOn.off  upper_bound=10 deg  lower_bound=-10 deg  hardstop_model=simscape.enum.hardstop.smooth  k_endstop=1e6 N*m/rad  D_endstop=10 N*m*s/rad  transition=0.001 rad  coeff_rest=0.7  w_tol_hardstop=0.1 rad/s  trq_tol=0.001 N*m  x0=0 deg
  Compliance ShaftR : sdl_lib/Couplings & Drives/Torsional Spring-Damper  k=1000*100 N*m/rad  mu_visc=1e3*10 N*m*s/rad  trq_coulomb=0 N*m  static_kinetic_ratio=1.1  w_tol=0.001 rad/s  model_hardstop=sdl.enum.hardStopOffOn.off  upper_bound=10 deg  lower_bound=-10 deg  hardstop_model=simscape.enum.hardstop.smooth  k_endstop=1e6 N*m/rad  D_endstop=10 N*m*s/rad  transition=0.001 rad  coeff_rest=0.7  w_tol_hardstop=0.1 rad/s  trq_tol=0.001 N*m  x0=0 deg
  Differential : sdl_lib/Gears/Differential  driveshaft_location=sdl.enum.differential_orientation.left  cd_ratio=1  friction_model=sdl.enum.gear_friction.none  efficiency=[.85, .92]  temperature_TLU=[280, 300, 320] K  efficiency_ss_TLU=[.95, .9, .85]  efficiency_cd_TLU=[.95, .9, .85]  pwr_thr=[.001, .001] W  mu_visc=[0, 0] N*m*s/rad  model_inertia=simscape.enum.onoff.off  sun_inertia=0.001 kg*m^2  sun_radius=0.01 m  carrier_inertia=0.001 kg*m^2  planet_inertia=0.001 kg*m^2  planet_mass=0.001 kg  thermal_mass=50 J/K  T_init=300 K
  Divide : Product  Inputs=*/
  Mechanical Rotational Reference : fl_lib/Mechanical/Rotational Elements/Mechanical Rotational Reference
  Mechanical Rotational Reference1 : fl_lib/Mechanical/Rotational Elements/Mechanical Rotational Reference
  Motor : Subsystem  Variant=on  VariantControlMode=label  VariantControl=Motor  LabelModeActiveChoice=Ideal  mask{popup_motor_type=Ideal}
      mask prompts: popup_motor_type "Motor Type"
      mask init:
      | bh = gcb;
      | motType = get_param(gcb,'popup_motor_type');
      | set_param(bh,'LabelModeActiveChoice',motType);
      settings: AttributesFormatString=%<popup_motor_type>
      mask TypeOptions popup_motor_type: Ideal | Electric
  Multibody InterfaceL : fl_lib/Mechanical/Multibody Interfaces/Rotational Multibody Interface
  Multibody InterfaceR : fl_lib/Mechanical/Multibody Interfaces/Rotational Multibody Interface
  Radius : Constant  Value=ForkliftParams.groundContact.frontTireRad
  Revolute Whl FL : sm_lib/Joints/Revolute Joint  JointMode=Normal  CompositeWrenchDir=FollowerOnBase  CompositeWrenchFrame=BaseFrame  SenseConstraintForce=off  SenseConstraintTorque=off  SenseTotalForce=off  SenseTotalTorque=off  PositionTargetSpecify=off  PositionTargetPriority=High  PositionTargetValue=0  PositionTargetValueUnits=deg  VelocityTargetSpecify=off  VelocityTargetPriority=High  VelocityTargetValue=0  VelocityTargetValueUnits=deg/s  EquilibriumPosition=0  EquilibriumPositionUnits=deg  SpringStiffness=0  SpringStiffnessUnits=N*m/deg  DampingCoefficient=0  DampingCoefficientUnits=N*m/(deg/s)  LowerLimitSpecify=off  LowerLimitBound=-90  LowerLimitBoundUnits=deg  LowerLimitStiffness=1e4  LowerLimitStiffnessUnits=N*m/deg  LowerLimitDamping=10  LowerLimitDampingUnits=N*m/(deg/s)  LowerLimitTransitionRegionWidth=0.1  LowerLimitTransitionRegionWidthUnits=deg  UpperLimitSpecify=off  UpperLimitBound=90  UpperLimitBoundUnits=deg  UpperLimitStiffness=1e4  UpperLimitStiffnessUnits=N*m/deg  UpperLimitDamping=10  UpperLimitDampingUnits=N*m/(deg/s)  UpperLimitTransitionRegionWidth=0.1  UpperLimitTransitionRegionWidthUnits=deg  TorqueActuationMode=InputTorque  MotionActuationMode=ComputedMotion  SensePosition=off  SenseVelocity=on  SenseAcceleration=off  SenseTorqueForce=off  SenseLowerLimitTorqueForce=off  SenseUpperLimitTorqueForce=off
  Revolute Whl FR : sm_lib/Joints/Revolute Joint  JointMode=Normal  CompositeWrenchDir=FollowerOnBase  CompositeWrenchFrame=BaseFrame  SenseConstraintForce=off  SenseConstraintTorque=off  SenseTotalForce=off  SenseTotalTorque=off  PositionTargetSpecify=off  PositionTargetPriority=High  PositionTargetValue=0  PositionTargetValueUnits=deg  VelocityTargetSpecify=off  VelocityTargetPriority=High  VelocityTargetValue=0  VelocityTargetValueUnits=deg/s  EquilibriumPosition=0  EquilibriumPositionUnits=deg  SpringStiffness=0  SpringStiffnessUnits=N*m/deg  DampingCoefficient=0  DampingCoefficientUnits=N*m/(deg/s)  LowerLimitSpecify=off  LowerLimitBound=-90  LowerLimitBoundUnits=deg  LowerLimitStiffness=1e4  LowerLimitStiffnessUnits=N*m/deg  LowerLimitDamping=10  LowerLimitDampingUnits=N*m/(deg/s)  LowerLimitTransitionRegionWidth=0.1  LowerLimitTransitionRegionWidthUnits=deg  UpperLimitSpecify=off  UpperLimitBound=90  UpperLimitBoundUnits=deg  UpperLimitStiffness=1e4  UpperLimitStiffnessUnits=N*m/deg  UpperLimitDamping=10  UpperLimitDampingUnits=N*m/(deg/s)  UpperLimitTransitionRegionWidth=0.1  UpperLimitTransitionRegionWidthUnits=deg  TorqueActuationMode=InputTorque  MotionActuationMode=ComputedMotion  SensePosition=off  SenseVelocity=on  SenseAcceleration=off  SenseTorqueForce=off  SenseLowerLimitTorqueForce=off  SenseUpperLimitTorqueForce=off
  Vis Fn L : sm_forklift_lib/Vis Fn  VariantControl=Vis Fn R  LabelModeActiveChoice=On  popup_fnVis_onOff=On  vis_offset=(ForkliftParams.groundContact.frontTireRad-0.02)
  Vis Fn R : sm_forklift_lib/Vis Fn  VariantControl=Vis Fn R  LabelModeActiveChoice=On  popup_fnVis_onOff=On  vis_offset=(ForkliftParams.groundContact.frontTireRad-0.02)
  Whl L : Subsystem
      mask Display: image('sm_forklift_wheelL_image.png')
  Whl R : Subsystem
      mask Display: image('sm_forklift_wheelR_image.png');
  Cha : PMIOPort  Side=Left
  Mast : PMIOPort  Port=2  Side=Right
  G : PMIOPort  Port=3  Side=Right
  Out Bus Element : Outport  PortName=Fn  Element=FL
  Out Bus Element2 : Outport  PortName=Fn  Element=FR
  Out Bus Element1 : Outport  Port=2  PortName=m  Element=vtFR
  Out Bus Element3 : Outport  Port=2  PortName=m  Element=vtFL
  wires:
  Radius/1 -> Divide/2
  Vel/1 -> Divide/1
  Whl L/1(FnO) -> Vis Fn L/1, Out Bus Element/1
  Whl R/1(FnO) -> Vis Fn R/1, Out Bus Element2/1
  Whl R/2(vt) -> Out Bus Element1/1
  Whl L/2(vt) -> Out Bus Element3/1
  Divide/1 -> Motor/1(w)
  connections:
  Differential/RConn2 -- Compliance ShaftL/LConn1
  Compliance ShaftL/RConn1 -- Multibody InterfaceL/LConn2
  Revolute Whl FL/RConn2 -- Multibody InterfaceL/RConn1
  Revolute Whl FL/LConn2 -- Multibody InterfaceL/LConn1
  Multibody InterfaceL/RConn2 -- Mechanical Rotational Reference/LConn1
  Multibody InterfaceR/RConn2 -- Mechanical Rotational Reference1/LConn1
  Revolute Whl FR/RConn2 -- Multibody InterfaceR/RConn1
  Revolute Whl FR/LConn2 -- Multibody InterfaceR/LConn1
  Compliance ShaftR/RConn1 -- Multibody InterfaceR/LConn2
  Compliance ShaftR/LConn1 -- Differential/RConn1
  Axle/LConn1 -- Cha/RConn1
  Axle/RConn1 -- Mast/RConn1
  Axle/RConn2 -- Vis Fn R/LConn1 -- Revolute Whl FR/LConn1
  G/RConn1 -- Whl R/RConn1 -- Whl L/RConn1
  Whl L/LConn1 -- Revolute Whl FL/RConn1
  Whl R/LConn1 -- Revolute Whl FR/RConn1
  Motor/RConn1 -- Differential/LConn1
  Revolute Whl FL/LConn1 -- Axle/LConn2 -- Vis Fn L/LConn1

== system sm_forklift/Forklift/AxleR ==
  Str : Inport
  Revolute Whl RL : sm_lib/Joints/Revolute Joint  JointMode=Normal  CompositeWrenchDir=FollowerOnBase  CompositeWrenchFrame=BaseFrame  SenseConstraintForce=off  SenseConstraintTorque=off  SenseTotalForce=off  SenseTotalTorque=off  PositionTargetSpecify=off  PositionTargetPriority=High  PositionTargetValue=0  PositionTargetValueUnits=deg  VelocityTargetSpecify=off  VelocityTargetPriority=High  VelocityTargetValue=0  VelocityTargetValueUnits=deg/s  EquilibriumPosition=0  EquilibriumPositionUnits=deg  SpringStiffness=0  SpringStiffnessUnits=N*m/deg  DampingCoefficient=0  DampingCoefficientUnits=N*m/(deg/s)  LowerLimitSpecify=off  LowerLimitBound=-90  LowerLimitBoundUnits=deg  LowerLimitStiffness=1e4  LowerLimitStiffnessUnits=N*m/deg  LowerLimitDamping=10  LowerLimitDampingUnits=N*m/(deg/s)  LowerLimitTransitionRegionWidth=0.1  LowerLimitTransitionRegionWidthUnits=deg  UpperLimitSpecify=off  UpperLimitBound=90  UpperLimitBoundUnits=deg  UpperLimitStiffness=1e4  UpperLimitStiffnessUnits=N*m/deg  UpperLimitDamping=10  UpperLimitDampingUnits=N*m/(deg/s)  UpperLimitTransitionRegionWidth=0.1  UpperLimitTransitionRegionWidthUnits=deg  TorqueActuationMode=NoTorque  MotionActuationMode=ComputedMotion  SensePosition=off  SenseVelocity=off  SenseAcceleration=off  SenseTorqueForce=off  SenseLowerLimitTorqueForce=off  SenseUpperLimitTorqueForce=off
  Revolute Whl RR : sm_lib/Joints/Revolute Joint  JointMode=Normal  CompositeWrenchDir=FollowerOnBase  CompositeWrenchFrame=BaseFrame  SenseConstraintForce=off  SenseConstraintTorque=off  SenseTotalForce=off  SenseTotalTorque=off  PositionTargetSpecify=off  PositionTargetPriority=High  PositionTargetValue=0  PositionTargetValueUnits=deg  VelocityTargetSpecify=off  VelocityTargetPriority=High  VelocityTargetValue=0  VelocityTargetValueUnits=deg/s  EquilibriumPosition=0  EquilibriumPositionUnits=deg  SpringStiffness=0  SpringStiffnessUnits=N*m/deg  DampingCoefficient=0  DampingCoefficientUnits=N*m/(deg/s)  LowerLimitSpecify=off  LowerLimitBound=-90  LowerLimitBoundUnits=deg  LowerLimitStiffness=1e4  LowerLimitStiffnessUnits=N*m/deg  LowerLimitDamping=10  LowerLimitDampingUnits=N*m/(deg/s)  LowerLimitTransitionRegionWidth=0.1  LowerLimitTransitionRegionWidthUnits=deg  UpperLimitSpecify=off  UpperLimitBound=90  UpperLimitBoundUnits=deg  UpperLimitStiffness=1e4  UpperLimitStiffnessUnits=N*m/deg  UpperLimitDamping=10  UpperLimitDampingUnits=N*m/(deg/s)  UpperLimitTransitionRegionWidth=0.1  UpperLimitTransitionRegionWidthUnits=deg  TorqueActuationMode=NoTorque  MotionActuationMode=ComputedMotion  SensePosition=off  SenseVelocity=off  SenseAcceleration=off  SenseTorqueForce=off  SenseLowerLimitTorqueForce=off  SenseUpperLimitTorqueForce=off
  Steering : Subsystem
      settings: PortSchema="{\"entries\":[{\"content\":{\"sides\":[{\"content\":{\"connectorIds\":[\"In1\",\"LConn1\"]},\"type\":\"ConnectorPlacement.EquallySpacedRectSide\",\"uuid\":\"0d510b34-ab99-44a4-a11b-984d94b4b900\"},{\"content\":{\"connectorIds\":[\"Out1\",\"RConn1\"],\"side\":\"RIGHT\"},\"type\":\"ConnectorPlacement.EquallySpacedRectSide\",\"uuid\":\"4c1d703c-01ab-4a3f-bf2a-9ce834e673e4\"},{\"content\":{\"connectorIds\":[\"LConn2\"],\"side\":\"TOP\"},\"type\":\"ConnectorPlacement.EquallySpacedRectSide\",\"uuid\":\"63dc5a65-cf73-4118-be0e-071c2cdc8991\"}]},\"type\":\"ConnectorPlacement.EquallySpacedConnector\",\"uuid\":\"f20c254a-232a-4385-850a-d1aaea4825d6\"}],\"packageUris\":[\"http://schema.mathworks.com/mf0/Connector/R2020b\"],\"version\":\"1.0\"}"
      mask Display: image('sm_forklift_axleRsteer_image.png')
  Vis Fn L : sm_forklift_lib/Vis Fn  VariantControl=Vis Fn R  LabelModeActiveChoice=On  popup_fnVis_onOff=On  vis_offset=(ForkliftParams.groundContact.rearTireRad-0.02)
  Vis Fn R : sm_forklift_lib/Vis Fn  VariantControl=Vis Fn R  LabelModeActiveChoice=On  popup_fnVis_onOff=On  vis_offset=(ForkliftParams.groundContact.rearTireRad-0.02)
  Whl RL : Subsystem
      mask Display: image('sm_forklift_wheelL_image.png')
  Whl RR : Subsystem
      mask Display: image('sm_forklift_wheelR_image.png')
  CW : PMIOPort  Side=Right
  G : PMIOPort  Port=2  Side=Left
  Out Bus Element : Outport  PortName=Fn  Element=RR
  Out Bus Element2 : Outport  PortName=Fn  Element=RL
  qStr : Outport  Port=2
  Out Bus Element1 : Outport  Port=3  PortName=m  Element=vtRR
  Out Bus Element3 : Outport  Port=3  PortName=m  Element=vtRL
  wires:
  Whl RR/1(FnOut) -> Vis Fn L/1, Out Bus Element/1
  Whl RL/1(FnOut) -> Vis Fn R/1, Out Bus Element2/1
  Whl RR/2(vt) -> Out Bus Element1/1
  Whl RL/2(vt) -> Out Bus Element3/1
  Str/1 -> Steering/1(Str)
  Steering/1(qStr) -> qStr/1
  connections:
  Whl RR/LConn1 -- Revolute Whl RR/RConn1
  Whl RR/RConn1 -- G/RConn1 -- Whl RL/RConn1
  Revolute Whl RL/RConn1 -- Whl RL/LConn1
  Revolute Whl RL/LConn1 -- Steering/LConn1 -- Vis Fn R/LConn1
  Revolute Whl RR/LConn1 -- Vis Fn L/LConn1 -- Steering/RConn1
  Steering/LConn2 -- CW/RConn1
